simulink model "Toma_datos_inv"  (R2019a)
settings: Solver=VariableStepAuto  StartTime=0.0  StopTime=9000  RelTol=1e-3
values from neighbouring files (symbols this model uses):
  Tm = 0.6    [ANFIS_inverso.m]    (also in Codigo_Inverso.m; Codigo_directo.m = 0.2)
settings Model: Creator=Alejoxbg  LastModifiedBy=Jose
settings DataIOCC: ReturnWorkspaceOutputs=off

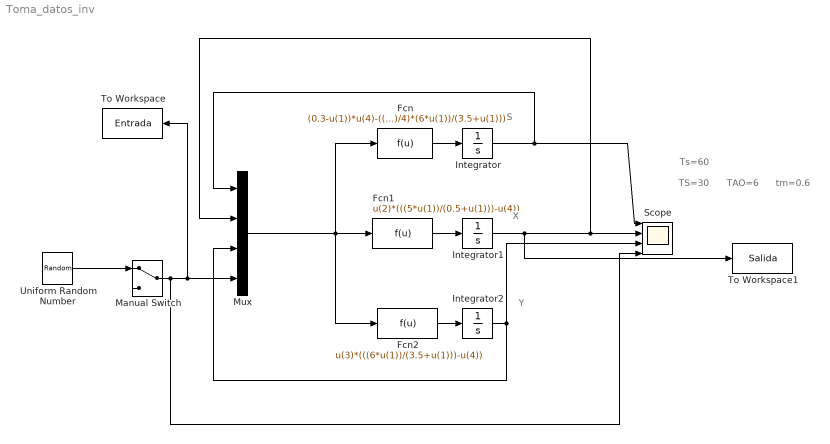
== system Toma_datos_inv ==
  note: TS=30
  note: tm=0.6
  note: TAO=6
  note: Ts=60
  note: S
  note: X
  note: Y
  Fcn : Fcn  Expr=(0.3-u(1))*u(4)-((u(2)/4)*(5*u(1))/(0.5+u(1)))-((u(3)/4)*(6*u(1))/(3.5+u(1)))
  Fcn1 : Fcn  Expr=u(2)*(((5*u(1))/(0.5+u(1)))-u(4))
  Fcn2 : Fcn  Expr=u(3)*(((6*u(1))/(3.5+u(1)))-u(4))
  Integrator : Integrator
  Integrator1 : Integrator  InitialCondition=0.1
  Integrator2 : Integrator
  Manual Switch : ManualSwitch
  Mux : Mux
  Scope : Scope  NumInputPorts=4
  To Workspace : ToWorkspace  VariableName=Entrada  SampleTime=Tm
  To Workspace1 : ToWorkspace  VariableName=Salida  SampleTime=Tm
  Uniform Random Number : UniformRandomNumber  Minimum=0.1  Maximum=1.7  Seed=456  SampleTime=60
  wires:
  Mux/1 -> Fcn/1, Fcn1/1, Fcn2/1
  Fcn1/1 -> Integrator1/1
  Integrator/1 -> Scope/1, Mux/1
  Integrator2/1 -> Mux/3, Scope/3
  Fcn/1 -> Integrator/1
  Manual Switch/1 -> Scope/4, Mux/4, To Workspace/1
  Integrator1/1 -> To Workspace1/1, Mux/2, Scope/2
  Fcn2/1 -> Integrator2/1
  Uniform Random Number/1 -> Manual Switch/1
